simulink model "nabludatel"  (R2021b)
settings: Solver=FixedStepAuto  StartTime=0.0  StopTime=0.5  FixedStep=Ts  RelTol=1e-3
values from neighbouring files (symbols this model uses):
  L = l'    [vipolnenie_lr_3.m]
  SYS = ss(a,b,c,d,Ts)    [vipolnenie_lr_3.m]
  Ts = 0.01    [vipolnenie_lr_3.m]
settings Model: Creator=Admin  LastModifiedBy=Admin

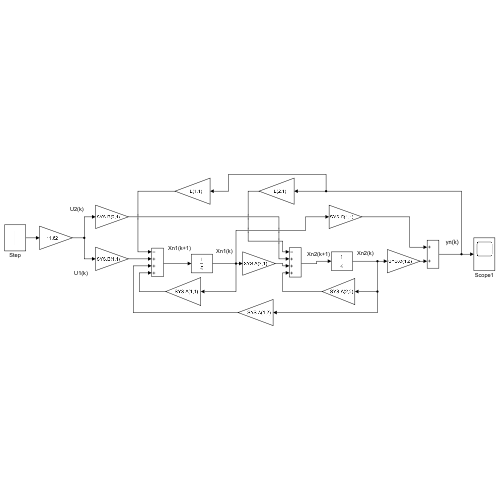
[thumbnail: Simulink's stored preview of the top-level diagram]
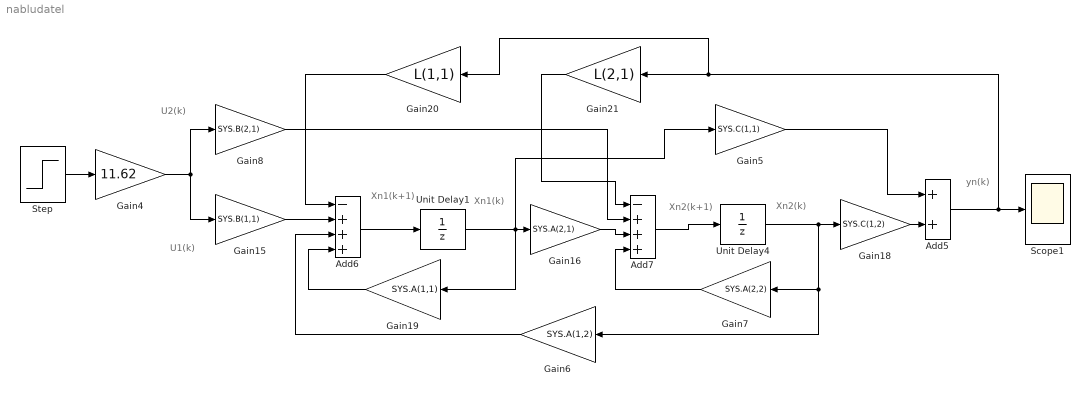
== system nabludatel ==
  note: Xn2(k)
  note: U2(k)
  note: Xn1(k)
  note: Xn2(k+1)
  note: U1(k)
  note: Xn1(k+1)
  note: yn(k)
  Add5 : Sum
  Add6 : Sum  Inputs=-+++
  Add7 : Sum  Inputs=-+++
  Gain15 : Gain  Gain=SYS.B(1,1)
  Gain16 : Gain  Gain=SYS.A(2,1)
  Gain18 : Gain  Gain=SYS.C(1,2)
  Gain19 : Gain  Gain=SYS.A(1,1)
  Gain20 : Gain  Gain=L(1,1)
  Gain21 : Gain  Gain=L(2,1)
  Gain4 : Gain  Gain=11.62
  Gain5 : Gain  Gain=SYS.C(1,1)
  Gain6 : Gain  Gain=SYS.A(1,2)
  Gain7 : Gain  Gain=SYS.A(2,2)
  Gain8 : Gain  Gain=SYS.B(2,1)
  Scope1 : Scope
  Step : Step  Time=0  SampleTime=0
  Unit Delay1 : UnitDelay  SampleTime=Ts  HasFrameUpgradeWarning=on
  Unit Delay4 : UnitDelay  SampleTime=Ts  HasFrameUpgradeWarning=on
  wires:
  Gain19/1 -> Add6/4
  Unit Delay1/1 -> Gain5/1, Gain19/1, Gain16/1
  Gain18/1 -> Add5/2
  Gain20/1 -> Add6/1
  Gain15/1 -> Add6/2
  Gain21/1 -> Add7/1
  Gain8/1 -> Add7/2
  Gain5/1 -> Add5/1
  Gain16/1 -> Add7/3
  Add6/1 -> Unit Delay1/1
  Gain6/1 -> Add6/3
  Add7/1 -> Unit Delay4/1
  Unit Delay4/1 -> Gain18/1, Gain7/1, Gain6/1
  Add5/1 -> Gain20/1, Gain21/1, Scope1/1
  Gain7/1 -> Add7/4
  Step/1 -> Gain4/1
  Gain4/1 -> Gain15/1, Gain8/1
